simulink model "AutomaticTransmission"  (R2020a)
settings: Solver=VariableStepAuto  StartTime=0.0  StopTime=10.0  RelTol=1e-3
values from neighbouring files (symbols this model uses):
  EngineMap = -40.0 215.0 245.0 264.0 264.0 267.0 267.0 267.0 267.0 267.0 -44.0 117.0 208.0 260.0 279.0 290.0 297.0 301.0 301.0 301.0 -49.0 85.0 178.0 241.0 282.0 293.0 305.0 308.0 312.0 312.0 -53.0 66.0 148.0 219.0 275.0 297.0 305.0 312.0 319.0 319.0 -57.0 44.0 122.0 193.0 260.0 290.0 305.0 319.0 327.0 327.0 -61.0 29.0 104.0 167.0 238.0 275.0 301.0 323.0 327.0 334.0 -65.0 10.0 85.0 152.0 223.0 260.0 293.0 319.    [DataDictionaryAutoTransmission.sldd]
  Iei = 0.0219914882835559    [DataDictionaryAutoTransmission.sldd]
  SpeedVector = 799.99999999999989 1200.0 1600.0 2000.0 2400.0 2800.0 3200.0 3600.0 4000.0 4400.0 4800.0    [DataDictionaryAutoTransmission.sldd]
  TorqueConvertorData = 0.0 0.1 0.2 0.3 0.4 0.5 0.6 0.7 0.8 0.81 0.82 0.83 0.84 0.85 0.86 0.87 0.88 0.89 0.9 0.92 0.94 137.4652089938063 137.065019156852 135.86444964598911 135.66435472751189 137.5652564530449 140.36658531172509 145.26891081441539 152.87251771654729 162.97731109964371 164.2779280697452 166.1788297952782 167.97968406157261 170.08068070558281 172.78196210502441 175.38319604522741 179.58518933324771 183.587    [DataDictionaryAutoTransmission.sldd]
  TorqueVector = 0.0 20.0 30.0 40.0 50.0 60.0 70.0 80.0 90.0 100.0    [DataDictionaryAutoTransmission.sldd]
  VehicleData = 3.23 40.0 0.02 1.0 12.094147857312469 0.0    [DataDictionaryAutoTransmission.sldd]
undefined symbols (not defined in the file or in its folder): downTable, downThresholdBP, sigbuilder_block, upTable, upThresholdBP
settings Model: DataDictionary=DataDictionaryAutoTransmission.sldd  Creator=DELL  LastModifiedBy=DELL

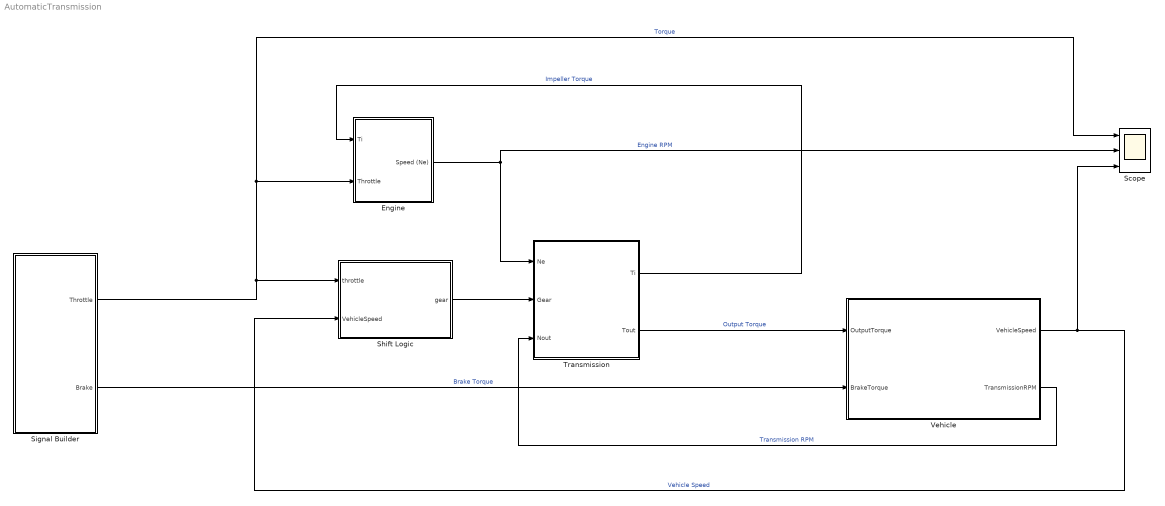
== system AutomaticTransmission ==
  Engine : Subsystem
  Scope : Scope  NumInputPorts=3
  Shift Logic : Stateflow chart  TreatAsAtomicUnit=on
  Signal Builder : Subsystem  Tag=STV Subsys  LoadFcn=sigbuilder_block('load');  StartFcn=sigbuilder_block('start');  StopFcn=sigbuilder_block('stop');  ClipboardFcn=sigbuilder_block('clipboard');  mask(Sigbuilder block){tuvar=[0:10]}
      mask help: Simulink:masks:SigbuilderBlock_MD
      mask init:
      | if ~strcmp(get_param(bdroot(gcbh),'SimulationStatus'),'stopped') tuvar = sigbuilder_block('maskInit'); end
      settings: CopyFcn=sigbuilder_block('copy');  DeleteFcn=sigbuilder_block('delete');  ModelCloseFcn=sigbuilder_block('modelClose');  PreSaveFcn=sigbuilder_block('preSave');  PauseFcn=sigbuilder_block('pause');  ContinueFcn=sigbuilder_block('continue');  NameChangeFcn=sigbuilder_block('namechange');  OpenFcn=sigbuilder_block('open',[437.6 199.2 550.4 400 ]);  CloseFcn=sigbuilder_block('close');
      mask Display: plot(0, 0, 100, 100,[2, 2, 32, 32, 2], [68, 8, 8, 68, 68],[32, 2], [38, 38], [32, 19, 2],[53, 60, 44], [32, 17, 17, 2],[16, 16, 31, 31]);txt = getActiveGroup(gcbh);text(2, 100, txt,'verticalAlignment', 'top');
  Transmission : Subsystem
  Vehicle : Subsystem  mask{Rfd=VehicleData(1), rload0=VehicleData(2), rload2=VehicleData(3), Rw=VehicleData(4), Iv=VehicleData(5), N20=VehicleData(6)/VehicleData(4)*VehicleData(1)}
      mask prompts: Rfd "Final Drive Ratio"; rload0 "Drag Friction at Wheels"; rload2 "Aerodynamic Drag"; Rw "Wheel Radius"; Iv "Vehicle Inertia"; N20 "Initial Transmission Output Speed"
      mask DialogControl DescGroupVar Prompt: Vehicle Parameters
      mask DialogControl DescTextVar Prompt: This subsystem shows how the vehicle behaves during different conditions.
  wires:
  Engine/1(Speed (Ne)) -> Scope/2, Transmission/1(Ne)  "Engine RPM"
  Shift Logic/1(gear) -> Transmission/2(Gear)
  Transmission/2(Tout) -> Vehicle/1(OutputTorque)  "Output Torque"
  Transmission/1(Ti) -> Engine/1(Ti)  "Impeller Torque"
  Vehicle/1(VehicleSpeed) -> Scope/3, Shift Logic/2(VehicleSpeed)  "Vehicle Speed"
  Signal Builder/1(Throttle) -> Scope/1, Engine/2(Throttle), Shift Logic/1(throttle)  "Torque"
  Signal Builder/2(Brake) -> Vehicle/2(BrakeTorque)  "Brake Torque"
  Vehicle/2(TransmissionRPM) -> Transmission/3(Nout)  "Transmission RPM"

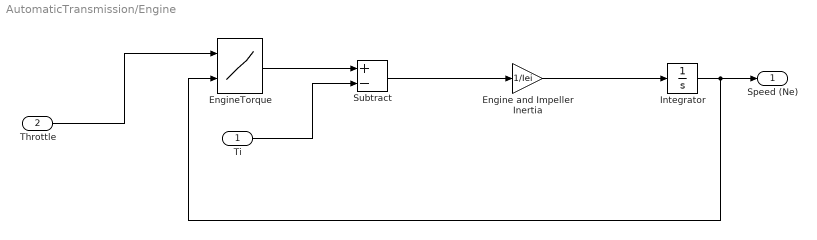
== system AutomaticTransmission/Engine ==
  Ti : Inport
  Throttle : Inport  Port=2
  "Engine and Impeller Inertia " : Gain  Gain=1/Iei
  EngineTorque : Lookup_n-D  BreakpointsForDimension1=TorqueVector  BreakpointsForDimension2=SpeedVector  Table=EngineMap  InputSameDT=on
  Integrator : Integrator  InitialCondition=1000  LimitOutput=on  UpperSaturationLimit=6000  LowerSaturationLimit=600  ZeroCross=off
  Subtract : Sum  Inputs=+-
  Speed (Ne) : Outport
  wires:
  Ti/1 -> Subtract/2
  Throttle/1 -> EngineTorque/1
  EngineTorque/1 -> Subtract/1
  Subtract/1 -> "Engine and Impeller Inertia "/1
  "Engine and Impeller Inertia "/1 -> Integrator/1
  Integrator/1 -> EngineTorque/2, Speed (Ne)/1

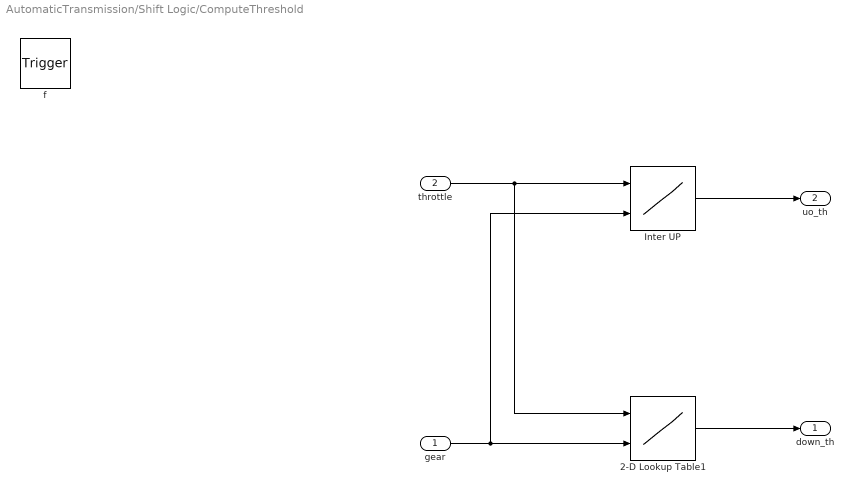
== system AutomaticTransmission/Shift Logic/ComputeThreshold ==
  gear : Inport  OutDataTypeStr=double  PortDimensions=1
  throttle : Inport  Port=2  OutDataTypeStr=double  PortDimensions=1
  f : TriggerPort  TriggerType=function-call  VariantControl=(inherit)
      settings: CopyFcn=Stateflow.SLINSF.SimulinkMan.removeBlockPreDeleteFcn  PreDeleteFcn=Stateflow.SLINSF.SimulinkMan.unsafePredeleteFcn
  2-D Lookup Table1 : Lookup_n-D  BreakpointsForDimension1=downThresholdBP  BreakpointsForDimension2=[1:4]  Table=downTable  InternalRulePriority=Speed  RndMeth=Simplest  InputSameDT=on
  Inter UP : Lookup_n-D  BreakpointsForDimension1=upThresholdBP  BreakpointsForDimension2=[1:4]  Table=upTable  InternalRulePriority=Speed  RndMeth=Simplest  InputSameDT=on
  down_th : Outport
  uo_th : Outport  Port=2
  wires:
  gear/1 -> Inter UP/2, 2-D Lookup Table1/2
  throttle/1 -> 2-D Lookup Table1/1, Inter UP/1
  Inter UP/1 -> uo_th/1
  2-D Lookup Table1/1 -> down_th/1

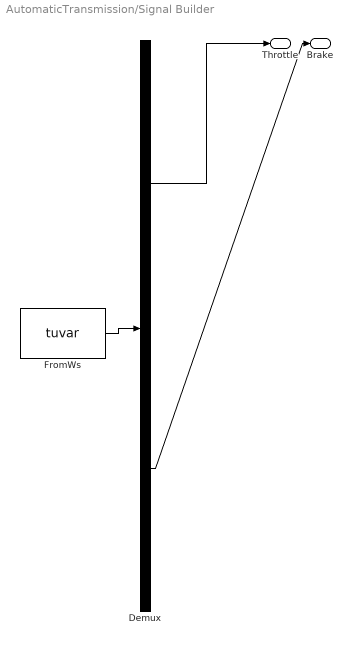
== system AutomaticTransmission/Signal Builder ==
  Demux : Demux  Tag=STV Demux  Outputs=2
      settings: DisplayOption=none
  FromWs : FromWorkspace  Tag=STV FromWs  VariableName=tuvar
      SigBuilderData=|
      | common.afterFinalStr = 'Extrapolate'
      | common.sampleTime = 0
      | dataSet.timeRange = [0 10]
      | dataSet.name = 'Group 1'
      | sbobj.Groups.Name = 'Group 1'
      | sbobj.Groups.Signals(1).Name = 'Throttle'
      | sbobj.Groups.Signals(1).XData = [0 4 4 6 6 10]
      | sbobj.Groups.Signals(1).YData = [0 0 1 1 0 0]
      | sbobj.Groups.Signals(2).Name = 'Brake'
      | sbobj.Groups.Signals(2).XData = [0 1 1 2 2 3 3 4 4 5 5 6 6 7 7 8 8 9 9 10]
      | sbobj.Groups.Signals(2).YData = [0 2 0 2 0 2 0 2 0 2 0 2 0 2 0 2 0 2 0 2]
  Throttle : Outport  Tag=STV Outport
  Brake : Outport  Tag=STV Outport  Port=2
  wires:
  Demux/1 -> Throttle/1
  FromWs/1 -> Demux/1
  Demux/2 -> Brake/1

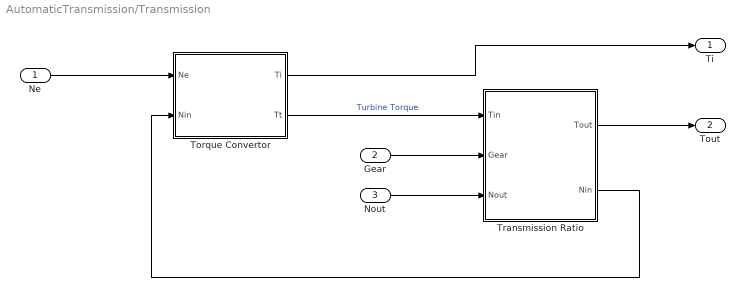
== system AutomaticTransmission/Transmission ==
  Ne : Inport
  Gear : Inport  Port=2
  Nout : Inport  Port=3
  Torque Convertor : Subsystem  mask{speedratio=TorqueConvertorData(:,1), Kfactor=TorqueConvertorData(:,2), Torkratio=TorqueConvertorData(:,3)}
      mask prompts: speedratio "Speed Ratio"; Kfactor "K Factor"; Torkratio "Torque Ratio"
      mask DialogControl DescGroupVar Prompt: Torque Convertor
      mask DialogControl DescTextVar Prompt: The values which are required for torque conversion are required.
  Transmission Ratio : Subsystem
  Ti : Outport
  Tout : Outport  Port=2
  wires:
  Transmission Ratio/1(Tout) -> Tout/1
  Torque Convertor/1(Ti) -> Ti/1
  Nout/1 -> Transmission Ratio/3(Nout)
  Torque Convertor/2(Tt) -> Transmission Ratio/1(Tin)  "Turbine Torque"
  Gear/1 -> Transmission Ratio/2(Gear)
  Transmission Ratio/2(Nin) -> Torque Convertor/2(Nin)
  Ne/1 -> Torque Convertor/1(Ne)

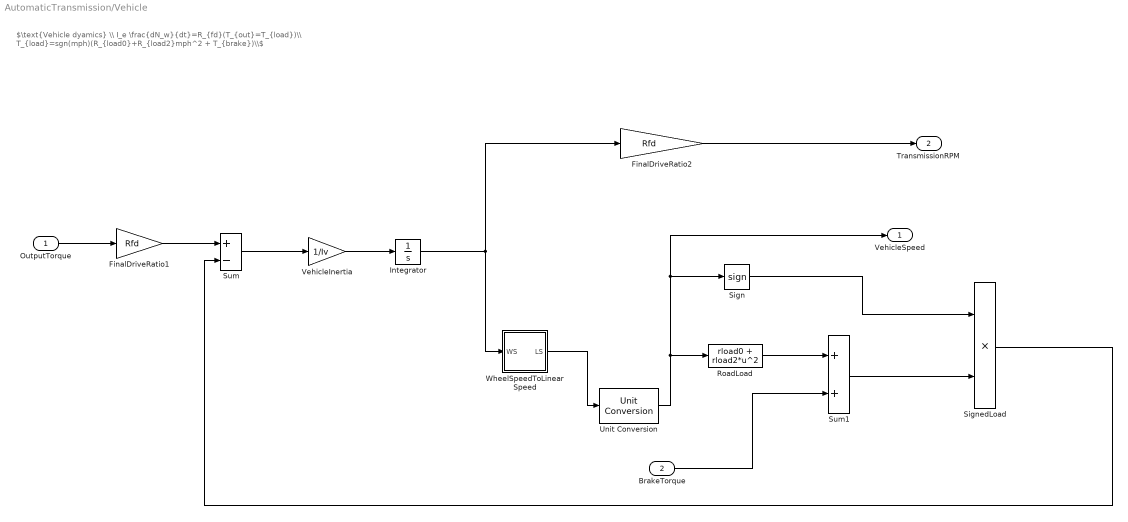
== system AutomaticTransmission/Vehicle ==
  note: $\text{Vehicle dyamics} \\ I_e \frac{dN_w}{dt}=R_{fd}(T_{out}=T_{load})\\ T_{load}=sgn(mph)(R_{load0}+R_{load2}mph^2 + T_{brake})\\$
  OutputTorque : Inport  Unit=ft*lbf@torque
  BrakeTorque : Inport  Port=2  Unit=ft*lbf@torque
  FinalDriveRatio1 : Gain  Gain=Rfd  SaturateOnIntegerOverflow=on  OutDataTypeStr=Inherit: Same as input  ParamDataTypeStr=Inherit: Same as input
  FinalDriveRatio2 : Gain  Gain=Rfd  SaturateOnIntegerOverflow=on  OutDataTypeStr=Inherit: Same as input  ParamDataTypeStr=Inherit: Same as input
  Integrator : Integrator
  RoadLoad : Fcn  Expr=rload0 + rload2*u^2
  Sign : Signum
  SignedLoad : Product  InputSameDT=on  SaturateOnIntegerOverflow=on  OutDataTypeStr=Inherit: Same as first input
  Sum : Sum  Inputs=+-  InputSameDT=on  SaturateOnIntegerOverflow=on  OutDataTypeStr=Inherit: Same as first input
  Sum1 : Sum  InputSameDT=on  SaturateOnIntegerOverflow=on  OutDataTypeStr=Inherit: Same as first input
  Unit Conversion : UnitConversion
  VehicleInertia : Gain  Gain=1/Iv  SaturateOnIntegerOverflow=on  OutDataTypeStr=Inherit: Same as input  ParamDataTypeStr=Inherit: Same as input
  WheelSpeedToLinearSpeed : Subsystem
  VehicleSpeed : Outport  Unit=mph  VectorParamsAs1DForOutWhenUnconnected=off
  TransmissionRPM : Outport  Port=2  Unit=rpm  VectorParamsAs1DForOutWhenUnconnected=off
  wires:
  Unit Conversion/1 -> VehicleSpeed/1, Sign/1, RoadLoad/1
  Sum/1 -> VehicleInertia/1
  SignedLoad/1 -> Sum/2
  VehicleInertia/1 -> Integrator/1
  OutputTorque/1 -> FinalDriveRatio1/1
  FinalDriveRatio2/1 -> TransmissionRPM/1
  Sum1/1 -> SignedLoad/2
  FinalDriveRatio1/1 -> Sum/1
  RoadLoad/1 -> Sum1/1
  BrakeTorque/1 -> Sum1/2
  Sign/1 -> SignedLoad/1
  Integrator/1 -> WheelSpeedToLinearSpeed/1(WS), FinalDriveRatio2/1
  WheelSpeedToLinearSpeed/1(LS) -> Unit Conversion/1

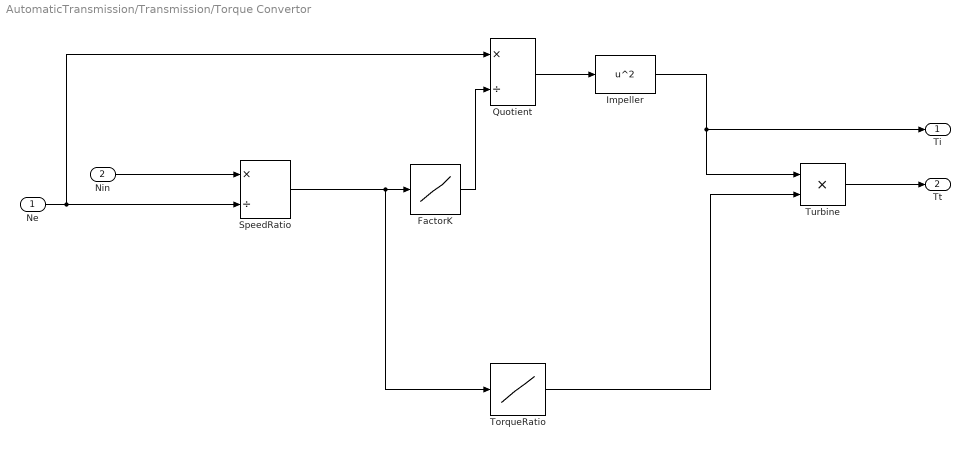
== system AutomaticTransmission/Transmission/Torque Convertor ==
  Ne : Inport
  Nin : Inport  Port=2
  FactorK : Lookup_n-D  NumberOfTableDimensions=1  BreakpointsForDimension1=speedratio  Table=Kfactor  SaturateOnIntegerOverflow=on  InputSameDT=on
  Impeller : Fcn  Expr=u^2
  Quotient : Product  Inputs=*/  InputSameDT=on  SaturateOnIntegerOverflow=on  OutDataTypeStr=Inherit: Same as first input
  SpeedRatio : Product  Inputs=*/  InputSameDT=on  SaturateOnIntegerOverflow=on  OutDataTypeStr=Inherit: Same as first input
  TorqueRatio : Lookup_n-D  NumberOfTableDimensions=1  BreakpointsForDimension1=speedratio  Table=Torkratio  SaturateOnIntegerOverflow=on  InputSameDT=on
  Turbine : Product  InputSameDT=on  SaturateOnIntegerOverflow=on  OutDataTypeStr=Inherit: Same as first input
  Ti : Outport  VectorParamsAs1DForOutWhenUnconnected=off
  Tt : Outport  Port=2  VectorParamsAs1DForOutWhenUnconnected=off
  wires:
  Nin/1 -> SpeedRatio/1
  Ne/1 -> SpeedRatio/2, Quotient/1
  Turbine/1 -> Tt/1
  Impeller/1 -> Turbine/1, Ti/1
  SpeedRatio/1 -> TorqueRatio/1, FactorK/1
  FactorK/1 -> Quotient/2
  Quotient/1 -> Impeller/1
  TorqueRatio/1 -> Turbine/2

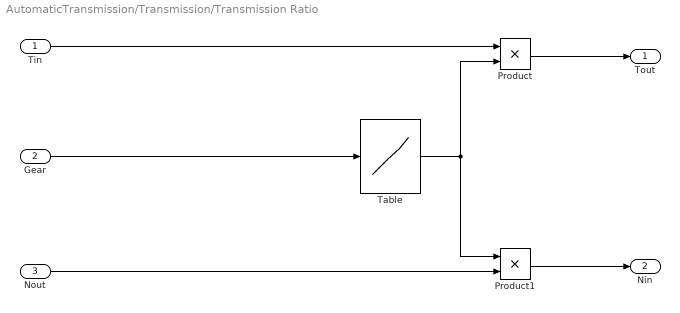
== system AutomaticTransmission/Transmission/Transmission Ratio ==
  Tin : Inport
  Gear : Inport  Port=2
  Nout : Inport  Port=3
  Product : Product
  Product1 : Product
  Table : Lookup_n-D  NumberOfTableDimensions=1  BreakpointsForDimension1=[1 2 3 4]  Table=[2.393 1.450 1.000 0.677]  OutDataTypeStr=double  SaturateOnIntegerOverflow=on  InputSameDT=on  LockScale=on
  Tout : Outport
  Nin : Outport  Port=2
  wires:
  Nout/1 -> Product1/2
  Tin/1 -> Product/1
  Gear/1 -> Table/1
  Table/1 -> Product1/1, Product/2
  Product/1 -> Tout/1
  Product1/1 -> Nin/1

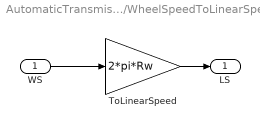
== system AutomaticTransmission/Vehicle/WheelSpeedToLinearSpeed ==
  WS : Inport  Unit=rpm
  ToLinearSpeed : Gain  Gain=2*pi*Rw  SaturateOnIntegerOverflow=on  OutDataTypeStr=Inherit: Same as input  ParamDataTypeStr=Inherit: Same as input
  LS : Outport  Unit=ft/min  VectorParamsAs1DForOutWhenUnconnected=off
  wires:
  ToLinearSpeed/1 -> LS/1
  WS/1 -> ToLinearSpeed/1

== stateflow chart AutomaticTransmission/Shift Logic ==
  state gear_state [parallel]
    settings: executionOrder=1
    state first
      en:
      gear = 1;
    state second
      en:
      gear = 2;
    state third
      en:
      gear = 3;
    state fourth
      en:
      gear = 4;
    (default) -> first
    second -> third [order 1] : up
    first -> second : up
    third -> fourth [order 1] : up
    third -> second [order 2] : down
    second -> first [order 2] : down
    fourth -> third : down
  state selectionState [parallel]
    during:
    [down_th up_th] = ComputeThreshold(gear,throttle);
    settings: executionOrder=2
    state SteadyState
    state DOWNshifting
    state UPshifting
    (default) -> SteadyState
    SteadyState -> DOWNshifting [order 2] : [VehicleSpeed < down_th]
    DOWNshifting -> SteadyState [order 2] : [VehicleSpeed > down_th]
    DOWNshifting -> SteadyState [order 1] : after(TWAIT,tick)
        | [VehicleSpeed <= down_th]
        | {gear_state.down}
    UPshifting -> SteadyState [order 1] : after(TWAIT,tick)
        | [VehicleSpeed >= up_th]
        | {gear_state.up}
    UPshifting -> SteadyState [order 2] : [VehicleSpeed < up_th]
    SteadyState -> UPshifting [order 1] : [VehicleSpeed > up_th]
  state [down_th,uo_th] = ComputeThreshold(gear,throttle) [function]
  (default) -> gear_state
  data: down_th function_output; uo_th function_output; gear function_input double size=1; throttle function_input double size=1; TWAIT parameter; down_th local; up_th local; throttle input; VehicleSpeed input; gear output
  events: up local FUNCTION_CALL_EVENT; down local FUNCTION_CALL_EVENT
